simulink library "UAVdesign_net"  (Simulink 7.7)
settings: Solver=ode45  SolverMode=SingleTasking  StartTime=0.0  StopTime=10.0  RelTol=1e-3
undefined symbols (not defined in the file or in its folder): alpha_IERA_IELA_IELA, R_IERA_RA_RA
libraries: UAVdesign_net x75, simulink x13
(part 8 of 8)

== matlab function Subsystem Models/Helicopter Rotor/Rotor Model (IERA)/Rotor Forces and Moments/Rotor Forces and Moments (Wind-Mast axes) ==
  data: Parameters input Bus: RotorParameters size=1; Environment input Bus: Environment size=1; FM_A output double size=6; va input double size=3; oma input double size=3; omid input double size=3; flap input double size=3; cz input double size=1; controls input double size=3; omega input double size=1; omegad input double size=1; FM_I output double size=6
function [FM_A, FM_I] = rotor_FM(Parameters, Environment, va, oma, omid, flap, cz, controls, omega, omegad)
% Modeling of the rotor forces and moments
% Implements equations 11.62, 11.63, 11.70, 11.71, 11.74
%   controls (3x1) = [theta0 A1 B1]' are the rotor control inputs
%   omega is the rotor rotation speed in body axes

bt = 1 - sqrt(2 * abs(cz)) / double(Parameters.nb);
bt = max([min([bt Parameters.btmax]) Parameters.btmin]);
sigma = double(Parameters.nb) * Parameters.chord / (pi * Parameters.radius);
if Parameters.iflap
    iflap = Parameters.iflap;
else
    iflap = Parameters.mbar * Parameters.radius^3 / 3;
end
clbar = -6 * cz / sigma;
cdavg = Parameters.del0_2(1) + clbar * (Parameters.del0_2(2) + clbar * Parameters.del0_2(3));
eps0 = cdavg / Parameters.a0;

bt2 = bt  * bt;
bt3 = bt2 * bt;
bt4 = bt3 * bt;
omegaa = omega - oma(3);
vtipa = omegaa * Parameters.radius;
mu = va(1) / vtipa;
mu2 = mu^2;
lambda = va(3) / vtipa;
pahat = oma(1) / omegaa;
qahat = oma(2) / omegaa;

fact1 = Environment.rho * pi * Parameters.radius^2 * vtipa^2;

% controls
theta0 = controls(1);
A1 = controls(2);
B1 = controls(3);
%flapping
beta0 = (flap(1) - Parameters.precone) * double(Parameters.hubtype) + Parameters.precone;
a1 = flap(2);
b1 = flap(3);

%   Find x-force
cxeps = bt2 * mu / 2;
cxth0 = bt * mu * lambda / 2 - bt3 * a1 / 3;
cxtht = bt2 * mu * lambda / 4 - bt4 * a1 / 4;
cxa1b1 = bt3 * beta0 / 6;
cxb1 = bt2 * lambda / 4 - bt2 * mu * a1 / 4;
cxlaa1 = 3 * bt2 / 4;
cxb02a12 = bt2 * mu / 4;
cxpa = bt3 * theta0 / 6 + bt4 * Parameters.twist / 8 + bt2 * lambda / 2;
cxpa = cxpa + 3 * bt2 * mu * B1 / 16 + bt2 * mu * a1 / 16;
cxqa = bt3 * beta0 / 6 + bt2 * mu * A1 / 16 + bt2 * mu * b1 / 16;
cx = -cxeps * eps0 + cxth0 * theta0 + cxtht * Parameters.twist + cxa1b1 * (A1 + b1);
cx = cx + cxb1 * B1 - cxlaa1 * lambda * a1 - cxb02a12 * (beta0 * beta0 + a1 * a1);
cx = cx + cxpa * pahat + cxqa * qahat;
cx = sigma * Parameters.a0 / 2 * cx;

%   Find y-force
cyth0 = (bt3 / 3 + bt * mu2 / 2) * b1 - 3 * bt2 * mu * beta0 / 4;
cytht = (bt4 / 4 + bt2 * mu2 / 4) * b1 - bt3 * mu * beta0 / 2;
cyca1 = bt2 * lambda / 4 + bt2 * mu * a1 / 4;
cycb1 = -(bt3 / 6 + bt * mu2 / 2) * beta0 + bt2 * mu * b1 / 2;
cyla = 3 * bt2 * b1 / 4 - 3 * bt * mu * beta0 / 2;
cya1 = bt3 * beta0 / 6 + bt2 * mu * b1 / 4 - bt * mu2 * beta0;
cypa = bt2 * mu * A1 / 16 - bt3 * beta0 / 6 + 5 * bt2 * mu * b1 / 16;
cyqa = bt3 * theta0 / 6 + bt4 * Parameters.twist / 8 + bt2 * lambda / 2 + bt2 * mu * B1 / 16 + 7 * bt2 * mu * a1 / 16;
cy = cyth0 * theta0 + cytht * Parameters.twist + cyca1 * A1 + cycb1 * B1;
cy = cy + cyla * lambda + cya1 * a1 + cypa * pahat + cyqa * qahat;
cy = sigma * Parameters.a0 / 2 * cy;

%   Find torque
if Parameters.btq
    bt = Parameters.btq;
    bt2 = bt  * bt;
    bt3 = bt2 * bt;
    bt4 = bt3 * bt;
end

cq0eps = bt4 / 4 + bt2 * mu2 / 4;
cq0la = bt3 * theta0 / 3 + bt4 * Parameters.twist / 4 + bt2 * lambda / 2;
cq0b02 = bt2 * mu2 / 4;
cq0a12 = bt4 / 8 + 3 * bt2 * mu2 / 16;
cq0b12 = bt4 / 8 + bt2 * mu2 / 16;
cq0b0b1 = bt3 * mu / 3;
cq0a1la = bt2 * mu / 2;
cq0 = cq0eps * eps0 - cq0la * lambda - cq0b02 * beta0 * beta0;
cq0 = cq0 - cq0a12 * a1 * a1 - cq0b12 * b1 * b1 + cq0b0b1 * beta0 * b1;
cq0 = cq0 - cq0a1la * a1 * lambda;
cq0 = sigma * Parameters.a0 / 2 * cq0;

cqcb1a1 = bt4 / 8 - bt2 * mu2 / 16;
cqcb1la = bt2 * mu / 4;
cqca1b0 = bt3 * mu / 6;
cqca1b1 = bt4 / 8 + bt2 * mu2 / 16;
cqcyc = cqcb1a1 * B1 * a1 - cqcb1la * B1 * lambda + cqca1b0 * A1 * beta0;
cqcyc = cqcyc - cqca1b1 * A1 * b1;
cqcyc = sigma * Parameters.a0 / 2 * cqcyc;

cqpa = -bt4 * B1 / 8 - bt3 * mu * theta0 / 6 - bt4 * mu * Parameters.twist / 8;
cqpa = cqpa - bt4 * pahat / 8 + bt4 * a1 / 4;
cqqa = -bt4 * A1 / 8 + bt3 * mu * beta0 / 3 - bt4 * qahat / 8 - bt4 * b1 / 4;
cqpq = cqpa * pahat + cqqa * qahat;
cqpq = sigma * Parameters.a0 / 2 * cqpq;

cq = cq0 + cqcyc + cqpq;

%   Get the hub loads
tork = cq * fact1 * Parameters.radius;
torki = double(Parameters.nb) * iflap * (omegad - omid(3));

FM_A = [ [cx; cy; cz]*fact1; [b1; a1]*Parameters.khub*double(Parameters.nb)/2; tork];
FM_I = [ 0; 0; 0; 0; 0; torki];

== matlab function Subsystem Models/Helicopter Rotor/Rotor Model (IERA)/Rotor Self-Influence/Rotor Wash Self-Influence (IERA) ==
  data: Parameters input Bus: RotorParameters size=1; Environment input Bus: Environment size=1; d output double size=3; va input double size=3; oma input double size=3; FM_A input double size=6
function d  = rotor_wash(Parameters, Environment, va, oma, FM_A)
% Rotor Self-Influence
% Implements the equation 12.4

vatot = sqrt(va' * va);
if vatot < 0.0001
    d = [0; 0; 0];
else
    rtworho = -1 / (2 * Environment.rho * vatot);
    a11 = 1 / (pi * Parameters.radius^2);
    a22 = a11;
    a33 = a11;
    d = rtworho * diag([a11 a22 a33]) * FM_A(1:3);
end

== matlab function Subsystem Models/Helicopter Rotor/Rotor Model (IERA)/Rotor Wash Iteration/Rotor Wash Iteration (Wind-Mast axes) ==
  data: Parameters input Bus: RotorParameters size=1; vi input double size=3; va_new output double size=3; va input double size=3; oma input double size=3; bt input double size=1; eps0 input double size=1; controls input double size=3; omega input double size=1; cz_new output double size=1; bt_new output double size=1; eps0_new output double size=1
function [va_new, cz_new, bt_new, eps0_new] = rotor_wash_iteration(Parameters, vi, va, oma, bt, eps0, controls, omega)
% Dynamic modeling of the rotor wake
% Implements the equation 11.119
%   controls (3x1) = [theta0 A1 B1]' are the rotor control inputs
%   omega is the rotor rotation speed in body axes
%   va (3x1), oma (3x1), bt, eps0 are initial conditions
%   d_dot is w_wash_dot

omegaa = omega - oma(3);
vtipa = omegaa * Parameters.radius;
mu = va(1) / vtipa;
mu2 = mu^2;
mu3 = mu^3;
lambda = va(3) / vtipa;
lambdi = vi(3) / vtipa;
lamw = lambdi - lambda;
pahat = oma(1) / omegaa;
theta0 = controls(1);
B1 = controls(3);
cz = 0;
sigma = double(Parameters.nb) * Parameters.chord / (pi * Parameters.radius);

dt = 2 * pi /omega / 10;
for i = 1:40,
    bt2 = bt  * bt;
    bt3 = bt2 * bt;
    bt4 = bt3 * bt;
    
    czth0 = bt3 / 3 + mu2 * bt / 2;
    cztht = bt4 / 4 + mu2 * bt2 / 4;
    czlam = (bt2 / 2 + mu2 / 4) * (1 + eps0);
    czcb1 = bt2 * mu / 2 + mu3 / 8;
    czpa = bt2 * mu / 4 * (1 + eps0);
    
    cz0 = czth0 * theta0 + cztht * Parameters.twist + czcb1 * B1 + czpa * pahat;
    cz0 = cz0 + czlam * lambda;
    cz  = -sigma * Parameters.a0 / 2 * cz0;
    
    fact2 = sqrt(mu^2 + lambda^2);
    lamwdot = 3 / 4 * omega * (-cz - 2 * fact2 * lamw);
    lamw = lamw + lamwdot * dt;
    lambda = lambdi - lamw;
    bt = 1 - sqrt(2 * abs(cz)) / double(Parameters.nb);
    bt = max([min([bt Parameters.btmax]) Parameters.btmin]);
    clbar = -6 * cz / sigma;
    cdavg = Parameters.del0_2(1) + clbar * (Parameters.del0_2(2) + clbar * Parameters.del0_2(3));
    eps0 = cdavg / Parameters.a0;
end

va(3) = lambda * vtipa;
cz_new = cz;
bt_new = bt;
eps0_new = eps0;
va_new = va;

== matlab function Subsystem Models/Helicopter Rotor/Rotor Model (IERA)/Wind-Mast Orientation/Wind Reference Axes ==
  data: VA_IERA input double size=3; T_WM_IERA output double size=[3 3]; T_IERA_WM output double size=[3 3]
function [T_WM_IERA,T_IERA_WM] = wind_mast(VA_IERA)

u = VA_IERA(1);
v = VA_IERA(2);

v_uv2 = u^2 + v^2;
if v_uv2 < 0.000001
    c3 = 1;
    s3 = 0;
else
    c3 = u / sqrt(v_uv2);
    s3 = v / sqrt(v_uv2);
end

s2 = 0;
c2 = 1;
c1 = 1;
s1 = 0;

T_WM_IERA = [c2*c3             c2*s3            -s2;   ...
            s1*s2*c3-c1*s3    s1*s2*s3+c1*c3   s1*c2; ...
            c1*s2*c3+s1*s3    c1*s2*s3-s1*c3   c1*c2];
T_IERA_WM = T_WM_IERA';

== matlab function Subsystem Models/Propeller/Rotor Forces and Moments (Inertial)/Rotor Forces and Moments (IERA) ==
  data: Parameters input Bus: PropellerParameters size=1; omi input double size=3; omega input double size=1; tau_motor input double size=1; FM_total output double size=6; FM_A input double size=6
function FM_total  = rotor_FM(Parameters, omi, omega, tau_motor, FM_A)
% Modeling of the rotor forces and moments
%   omega is the rotor rotation speed in body axes

if Parameters.iflap
    iflap = Parameters.iflap;
else
    iflap = Parameters.mbar * Parameters.radius^3 / 3;
end

if bitand(Parameters.flags, uint32(1))
    tau_motor = FM_A(6);
end
FM_total = [FM_A(1:5); 0] + [ 0; 0; 0; (double(Parameters.nb) * iflap)*omega*[omi(2); omi(1)]; tau_motor];

== matlab function Subsystem Models/Propeller/Rotor Model (IERA)/Rotor Forces and Moments (Aero)/Rotor Forces and Moments (Wind-Mast axes) ==
  data: Parameters input Bus: PropellerParameters size=1; Environment input Bus: Environment size=1; FM_A output double size=6; va input double size=3; oma input double size=3; cz input double size=1; controls input double size=1; omega input double size=1
function FM_A  = rotor_FM(Parameters, Environment, va, oma, cz, controls, omega)
% Modeling of the rotor forces and moments
% Implements equations 11.62, 11.63, 11.70, 11.71, 11.74
%   controls (3x1) = [theta0 A1 B1]' are the rotor control inputs
%   omega is the rotor rotation speed in body axes

bt = 1 - sqrt(2 * abs(cz)) / double(Parameters.nb);
bt = max([min([bt Parameters.btmax]) Parameters.btmin]);
sigma = double(Parameters.nb) * Parameters.chord / (pi * Parameters.radius);
clbar = -6 * cz / sigma;
cdavg = Parameters.del0_2(1) + clbar * (Parameters.del0_2(2) + clbar * Parameters.del0_2(3));
eps0 = cdavg / Parameters.a0;

bt2 = bt  * bt;
bt3 = bt2 * bt;
bt4 = bt3 * bt;
omegaa = omega - oma(3);
vtipa = omegaa * Parameters.radius;
mu = va(1) / vtipa;
mu2 = mu^2;
lambda = va(3) / vtipa;
pahat = oma(1) / omegaa;
qahat = oma(2) / omegaa;

fact1 = Environment.rho * pi * Parameters.radius^2 * vtipa^2;

% controls
theta0 = controls(1);

%   Find x-force
cxeps = bt2 * mu / 2;
cxth0 = bt * mu * lambda / 2;
cxtht = bt2 * mu * lambda / 4;
cxpa = bt3 * theta0 / 6 + bt4 * Parameters.twist / 8 + bt2 * lambda / 2;
cxqa = 0;
cx = -cxeps * eps0 + cxth0 * theta0 + cxtht * Parameters.twist;
cx = cx + cxpa * pahat + cxqa * qahat;
cx = sigma * Parameters.a0 / 2 * cx;

%   Find y-force
cyth0 = 0;
cytht = 0;
cyla = 0;
cypa = 0;
cyqa = bt3 * theta0 / 6 + bt4 * Parameters.twist / 8 + bt2 * lambda / 2;
cy = cyth0 * theta0 + cytht * Parameters.twist;
cy = cy + cyla * lambda + cypa * pahat + cyqa * qahat;
cy = sigma * Parameters.a0 / 2 * cy;


if Parameters.btq
    bt = Parameters.btq;
    bt2 = bt  * bt;
    bt3 = bt2 * bt;
    bt4 = bt3 * bt;
end

%   Find x-moment
cmx = - bt3 * mu / 3 * theta0 - bt4 * mu / 4 * Parameters.twist;
cmx = cmx - bt2 * mu / 4 * lambda - bt4 / 8 * pahat;
cmx = sigma * Parameters.a0 / 2 * cmx;

%   Find y-moment
cmy = - bt4 / 8 * qahat;
cmy = sigma * Parameters.a0 / 2 * cmy;

%   Find torque
cq0eps = bt4 / 4 + bt2 * mu2 / 4;
cq0la = bt3 * theta0 / 3 + bt4 * Parameters.twist / 4 + bt2 * lambda / 2;
cq0 = cq0eps * eps0 - cq0la * lambda;
cq0 = sigma * Parameters.a0 / 2 * cq0;

cqcyc = 0;
cqcyc = sigma * Parameters.a0 / 2 * cqcyc;

cqpa = - bt3 * mu * theta0 / 6 - bt4 * mu * Parameters.twist / 8;
cqpa = cqpa - bt4 * pahat / 8;
cqqa = - bt4 * qahat / 8;
cqpq = cqpa * pahat + cqqa * qahat;
cqpq = sigma * Parameters.a0 / 2 * cqpq;

cq = cq0 + cqcyc + cqpq;

%   Get the hub loads
FM_A = [ [cx; cy; cz]; Parameters.radius*[cmx; cmy; cq] ] * fact1;

== matlab function Subsystem Models/Propeller/Rotor Model (IERA)/Rotor Self-Influence/Rotor Wash Self-Influence (IERA) ==
  data: Parameters input Bus: PropellerParameters size=1; Environment input Bus: Environment size=1; d output double size=3; va input double size=3; oma input double size=3; FM_A input double size=6
function d  = rotor_wash(Parameters, Environment, va, oma, FM_A)
% Rotor Self-Influence
% Implements the equation 12.4

vatot = sqrt(va' * va);
if vatot < 0.0001
    d = [0; 0; 0];
else
    rtworho = -1 / (2 * Environment.rho * vatot);
    a11 = 1 / (pi * Parameters.radius^2);
    a22 = a11;
    a33 = a11;
    d = rtworho * diag([a11 a22 a33]) * FM_A(1:3);
end

== matlab function Subsystem Models/Propeller/Rotor Model (IERA)/Rotor Wash Iteration/Rotor Wash Iteration (Wind-Mast axes) ==
  data: Parameters input Bus: PropellerParameters size=1; vi input double size=3; va_new output double size=3; va input double size=3; oma input double size=3; bt input double size=1; eps0 input double size=1; controls input double size=1; omega input double size=1; cz_new output double size=1; bt_new output double size=1; eps0_new output double size=1
function [va_new, cz_new, bt_new, eps0_new] = rotor_wash_iteration(Parameters, vi, va, oma, bt, eps0, controls, omega)
% Dynamic modeling of the rotor wake
% Implements the equation 11.119
%   controls (3x1) = [theta0 A1 B1]' are the rotor control inputs
%   omega is the rotor rotation speed in body axes
%   va (3x1), oma (3x1), bt, eps0 are initial conditions
%   d_dot is w_wash_dot

omegaa = omega - oma(3);
vtipa = omegaa * Parameters.radius;
mu = va(1) / vtipa;
mu2 = mu^2;
lambda = va(3) / vtipa;
lambdi = vi(3) / vtipa;
lamw = lambdi - lambda;
pahat = oma(1) / omegaa;
theta0 = controls(1);
cz = 0;
sigma = double(Parameters.nb) * Parameters.chord / (pi * Parameters.radius);

dt = 2 * pi /omega / 10;
for i = 1:20,
    bt2 = bt  * bt;
    bt3 = bt2 * bt;
    bt4 = bt3 * bt;
    
    czth0 = bt3 / 3 + mu2 * bt / 2;
    cztht = bt4 / 4 + mu2 * bt2 / 4;
    czlam = (bt2 / 2 + mu2 / 4) * (1 + eps0);
    czpa = bt2 * mu / 4 * (1 + eps0);
    
    cz0 = czth0 * theta0 + cztht * Parameters.twist + czpa * pahat;
    cz0 = cz0 + czlam * lambda;
    cz  = -sigma * Parameters.a0 / 2 * cz0;
    
    fact2 = sqrt(mu^2 + lambda^2);
    lamwdot = 3 / 4 * omega * (-cz - 2 * fact2 * lamw);
    lamw = lamw + lamwdot * dt;
    lambda = lambdi - lamw;
    bt = 1 - sqrt(2 * abs(cz)) / double(Parameters.nb);
    bt = max([min([bt Parameters.btmax]) Parameters.btmin]);
    clbar = -6 * cz / sigma;
    cdavg = Parameters.del0_2(1) + clbar * (Parameters.del0_2(2) + clbar * Parameters.del0_2(3));
    eps0 = cdavg / Parameters.a0;
end

va(3) = lambda * vtipa;
cz_new = cz;
bt_new = bt;
eps0_new = eps0;
va_new = va;

== matlab function Subsystem Models/Propeller/Rotor Model (IERA)/Wind-Mast Orientation/Wind Reference Axes ==
  data: VA_IERA input double size=3; T_WM_IERA output double size=[3 3]; T_IERA_WM output double size=[3 3]
function [T_WM_IERA,T_IERA_WM] = wind_mast(VA_IERA)

u = VA_IERA(1);
v = VA_IERA(2);

v_uv2 = u^2 + v^2;
if v_uv2 < 0.000001
    c3 = 1;
    s3 = 0;
else
    c3 = u / sqrt(v_uv2);
    s3 = v / sqrt(v_uv2);
end

s2 = 0;
c2 = 1;
c1 = 1;
s1 = 0;

T_WM_IERA = [c2*c3             c2*s3            -s2;   ...
            s1*s2*c3-c1*s3    s1*s2*s3+c1*c3   s1*c2; ...
            c1*s2*c3+s1*s3    c1*s2*s3-s1*c3   c1*c2];
T_IERA_WM = T_WM_IERA';

== matlab function Subsystem Models/Propeller Rotation Dynamics/Propeller rotation dynamics ==
  data: Parameters input Bus: PropellerParameters size=1; omi input double size=3; omid input double size=3; omega input double size=1; tau_motor input double size=1; omegad output double; tau_prop input double size=1
function omegad  = rot_dyn(Parameters, omi, omid, omega, tau_motor, tau_prop)
% Modeling of the rotor forces and moments
%   omega is the rotor rotation speed in body axes

if Parameters.iflap
    iflap = Parameters.iflap;
else
    iflap = Parameters.mbar * Parameters.radius^3 / 3;
end

omegad = (tau_motor - tau_prop) / (double(Parameters.nb) * iflap) + omid(3);

== matlab function Subsystem Models/Wing/Wing Model (IERA)/Left Wing/Half Wing Forces and Moments/Wing Forces and Moments (WRA axes) ==
  data: Parameters input Bus: FinParameters size=1; Environment input Bus: Environment size=1; FM_A output double size=6; va input double size=3; oma input double size=3
function FM_A  = wing_FM(Parameters, Environment, va, oma)
% Modeling of the wing forces and moments

%   Calculate some intermediate wing constants.
slambda = Parameters.taper;
b = Parameters.span;
croot = Parameters.chord;
s12 = b * croot * (1 + slambda) / 4;
stot = s12 * 2;
cbar = 2 * croot * (slambda^2 + slambda + 1) / 3 / (slambda + 1);
ar = b^2 / stot;
a03d_coef = ar / (ar + 2 * (ar + 4) / (ar + 2));

%   Calculate aerodynamic loads in WRA
aoa = atan2(va(3), va(1));

a = aoa - fix(aoa/pi)*pi;
if a > pi/2
    a = -pi+a;
end
if a < -pi/2
    a = pi+a;
end
if abs(a) > Parameters.stall + 5*pi/180
    cl = Parameters.a1s2 * sin(2*a);
elseif abs(a) >=Parameters. stall
    k = (abs(a) - Parameters.stall) / (5*pi/180);
    cl = (1-k) * Parameters.a0 * a  + k * Parameters.a1s2 * sin(2*a);
else
    cl = Parameters.a0 * a;
end
cl = a03d_coef * cl;

cd = Parameters.cd0 + Parameters.cd1s1 * sin(aoa) + Parameters.cd2c1 * cos(aoa)^2;
cm = Parameters.cm0 + Parameters.cm1s1 * sin(aoa);

v2 = va'*va;
qtots12 = Environment.rho * v2 / 2 * s12;
drag = qtots12 * cd;
lift = qtots12 * cl;
momy = qtots12 * cbar * cm;
F = [-drag; 0; -lift];
M = [0; momy; 0];
Tt = [ cos(-aoa) 0 -sin(-aoa); 0 1 0; sin(-aoa) 0 cos(-aoa)];
FM_A = [Tt' * F; Tt' * M];

== matlab function Subsystem Models/Wing/Wing Model (IERA)/Right Wing/Half Wing Forces and Moments/Wing Forces and Moments (WRA axes) ==
  data: Parameters input Bus: FinParameters size=1; Environment input Bus: Environment size=1; FM_A output double size=6; va input double size=3; oma input double size=3
function FM_A  = wing_FM(Parameters, Environment, va, oma)
% Modeling of the wing forces and moments

%   Calculate some intermediate wing constants.
slambda = Parameters.taper;
b = Parameters.span;
croot = Parameters.chord;
s12 = b * croot * (1 + slambda) / 4;
stot = s12 * 2;
cbar = 2 * croot * (slambda^2 + slambda + 1) / 3 / (slambda + 1);
ar = b^2 / stot;
a03d_coef = ar / (ar + 2 * (ar + 4) / (ar + 2));

%   Calculate aerodynamic loads in WRA
aoa = atan2(va(3), va(1));

a = aoa - fix(aoa/pi)*pi;
if a > pi/2
    a = -pi+a;
end
if a < -pi/2
    a = pi+a;
end
if abs(a) > Parameters.stall + 5*pi/180
    cl = Parameters.a1s2 * sin(2*a);
elseif abs(a) >=Parameters. stall
    k = (abs(a) - Parameters.stall) / (5*pi/180);
    cl = (1-k) * Parameters.a0 * a  + k * Parameters.a1s2 * sin(2*a);
else
    cl = Parameters.a0 * a;
end
cl = a03d_coef * cl;

cd = Parameters.cd0 + Parameters.cd1s1 * sin(aoa) + Parameters.cd2c1 * cos(aoa)^2;
cm = Parameters.cm0 + Parameters.cm1s1 * sin(aoa);

v2 = va'*va;
qtots12 = Environment.rho * v2 / 2 * s12;
drag = qtots12 * cd;
lift = qtots12 * cl;
momy = qtots12 * cbar * cm;
F = [-drag; 0; -lift];
M = [0; momy; 0];
Tt = [ cos(-aoa) 0 -sin(-aoa); 0 1 0; sin(-aoa) 0 cos(-aoa)];
FM_A = [Tt' * F; Tt' * M];

== matlab function Subsystem Models/Wing/Wing Model (IERA)/Wing Self-Influence/Wing Wash Self-Influence (IERA ==
  data: Parameters input Bus: FinParameters size=1; Environment input Bus: Environment size=1; d output double size=3; va input double size=3; oma input double size=3; FM_A input double size=6
function d  = wing_wash(Parameters, Environment, va, oma, FM_A)
% Wing Self-Influence
% Implements the equation 12.12

vatot = sqrt(va' * va);
if vatot < 0.0001
    d = [0; 0; 0];
else
    rtworho = -1 / (2 * Environment.rho * vatot);
    a11 = 4 / (pi * Parameters.span^2);
    a22 = a11;
    a33 = a11;
    d = rtworho * diag([a11 a22 a33]) * FM_A(1:3);
end
